simulink model "building_EXAMPLE_v1"  (R2016b)
settings: Solver=ode23tb  StartTime=-building.preruntime+8760*3600  StopTime=building.runtime+8760*3600  MaxStep=600  EnableMultiTasking=on
StartFcn:
  | tic
StopFcn:
  | toc
values from neighbouring files (symbols this model uses):
  building = create_building_automatic(building, modify, import_mode, name_XML, name_EXCEL, name_PHPP, NUMBEROFZONES)    [work_EXAMPLE_v1.m]
undefined symbols (not defined in the file or in its folder): A, B, C, cp, Dd, Dreifach, FluidMix, get_building, ID, MassFlow, p, Pressure, Qdot_C, Qdot_C_energy, Qdot_H, Qdot_H_energy, Qdot_I_electricity, Qdot_I_electricity_energy, Qdot_I_light, Qdot_I_light_energy, Qdot_I_person, Qdot_I_person_energy, Qdot_S, Qdot_S_energy, Qdot_T_ground, Qdot_T_ground_energy, Qdot_T_neighbour, Qdot_T_neighbour_energy, Qdot_T_opaque, Qdot_T_opaque_energy, Qdot_T_window, Qdot_T_window_energy, Qdot_V_infiltration, Qdot_V_infiltration_energy, Qdot_V_mech, Qdot_V_mech_energy, Qdot_V_window, Qdot_V_window_energy, rho, Tc, Temperature, Tr, Ts, Wärmeschutzglas, x_CO2, x_H2O, x_VOC
libraries: carnotUIBK x1931, carnot x83, simulink_extras x22, simulink x12
(part 34 of 35)

== system building_EXAMPLE_v1/DATALOGGER/logger_BDB/z5 ==
  BDB : Inport
  Bus Assignment : BusAssignment  AssignedSignals=Qdot_T_opaque_energy,Qdot_T_ground_energy,Qdot_T_neighbour_energy,Qdot_T_window_energy,Qdot_V_mech_energy,Qdot_V_window_energy,Qdot_V_infiltration_energy,Qdot_S_energy,Qdot_I_person_energy,Qdot_I_light_energy,Qdot_I_electricity_energy,Qdot_H_energy,Qdot_C_energy
  Bus Creator1 : BusCreator  Inputs=13
  Bus Selector1 : BusSelector  OutputSignals=z5.Qdot_T_opaque,z5.Qdot_T_ground,z5.Qdot_T_neighbour,z5.Qdot_T_window,z5.Qdot_V_mech,z5.Qdot_V_window,z5.Qdot_V_infiltration,z5.Qdot_S,z5.Qdot_I_person,z5.Qdot_I_light,z5.Qdot_I_electricity,z5.Qdot_H,z5.Qdot_C
  Constant{,1..12} (13 alike) : Constant  Value=0
  Subsystem : Subsystem
  Subsystem1 : Subsystem
  Subsystem10 : Subsystem
  Subsystem11 : Subsystem
  Subsystem12 : Subsystem
  Subsystem2 : Subsystem
  Subsystem3 : Subsystem
  Subsystem4 : Subsystem
  Subsystem5 : Subsystem
  Subsystem6 : Subsystem
  Subsystem7 : Subsystem
  Subsystem8 : Subsystem
  Subsystem9 : Subsystem
  BDBenergy : Outport
  wires:
  Constant12/1 -> Bus Creator1/13  "Qdot_C_energy"
  Constant2/1 -> Bus Creator1/3  "Qdot_T_neighbour_energy"
  Constant4/1 -> Bus Creator1/5  "Qdot_V_mech_energy"
  Constant9/1 -> Bus Creator1/10  "Qdot_I_light_energy"
  Constant1/1 -> Bus Creator1/2  "Qdot_T_ground_energy"
  Constant3/1 -> Bus Creator1/4  "Qdot_T_window_energy"
  Constant11/1 -> Bus Creator1/12  "Qdot_H_energy"
  Constant10/1 -> Bus Creator1/11  "Qdot_I_electricity_energy"
  Constant/1 -> Bus Creator1/1  "Qdot_T_opaque_energy"
  Constant8/1 -> Bus Creator1/8  "Qdot_S_energy"
  Constant7/1 -> Bus Creator1/9  "Qdot_I_person_energy"
  Constant6/1 -> Bus Creator1/7  "Qdot_V_infiltration_energy"
  BDB/1 -> Bus Selector1/1
  Constant5/1 -> Bus Creator1/6  "Qdot_V_window_energy"
  Bus Selector1/1 -> Subsystem/1(In1)  "<Qdot_T_opaque>"
  Bus Selector1/4 -> Subsystem3/1(In1)  "<Qdot_T_window>"
  Bus Selector1/3 -> Subsystem2/1(In1)  "<Qdot_T_neighbour>"
  Bus Selector1/2 -> Subsystem1/1(In1)  "<Qdot_T_ground>"
  Bus Selector1/9 -> Subsystem8/1(In1)  "<Qdot_I_person>"
  Bus Selector1/10 -> Subsystem9/1(In1)  "<Qdot_I_light>"
  Bus Selector1/11 -> Subsystem10/1(In1)  "<Qdot_I_electricity>"
  Bus Selector1/12 -> Subsystem11/1(In1)  "<Qdot_H>"
  Bus Selector1/13 -> Subsystem12/1(In1)  "<Qdot_C>"
  Bus Selector1/8 -> Subsystem7/1(In1)  "<Qdot_S>"
  Bus Selector1/7 -> Subsystem6/1(In1)  "<Qdot_V_infiltration>"
  Bus Selector1/6 -> Subsystem5/1(In1)  "<Qdot_V_window>"
  Bus Selector1/5 -> Subsystem4/1(In1)  "<Qdot_V_mech>"
  Bus Assignment/1 -> BDBenergy/1
  Bus Creator1/1 -> Bus Assignment/1
  Subsystem/1(Out1) -> Bus Assignment/2
  Subsystem12/1(Out1) -> Bus Assignment/14
  Subsystem11/1(Out1) -> Bus Assignment/13
  Subsystem10/1(Out1) -> Bus Assignment/12
  Subsystem9/1(Out1) -> Bus Assignment/11
  Subsystem8/1(Out1) -> Bus Assignment/10
  Subsystem7/1(Out1) -> Bus Assignment/9
  Subsystem6/1(Out1) -> Bus Assignment/8
  Subsystem5/1(Out1) -> Bus Assignment/7
  Subsystem4/1(Out1) -> Bus Assignment/6
  Subsystem3/1(Out1) -> Bus Assignment/5
  Subsystem2/1(Out1) -> Bus Assignment/4
  Subsystem1/1(Out1) -> Bus Assignment/3

== system building_EXAMPLE_v1/DATALOGGER/logger_BDB/z6 ==
  BDB : Inport
  Bus Assignment : BusAssignment  AssignedSignals=Qdot_T_opaque_energy,Qdot_T_ground_energy,Qdot_T_neighbour_energy,Qdot_T_window_energy,Qdot_V_mech_energy,Qdot_V_window_energy,Qdot_V_infiltration_energy,Qdot_S_energy,Qdot_I_person_energy,Qdot_I_light_energy,Qdot_I_electricity_energy,Qdot_H_energy,Qdot_C_energy
  Bus Creator1 : BusCreator  Inputs=13
  Bus Selector1 : BusSelector  OutputSignals=z6.Qdot_T_opaque,z6.Qdot_T_ground,z6.Qdot_T_neighbour,z6.Qdot_T_window,z6.Qdot_V_mech,z6.Qdot_V_window,z6.Qdot_V_infiltration,z6.Qdot_S,z6.Qdot_I_person,z6.Qdot_I_light,z6.Qdot_I_electricity,z6.Qdot_H,z6.Qdot_C
  Constant{,1..12} (13 alike) : Constant  Value=0
  Subsystem : Subsystem
  Subsystem1 : Subsystem
  Subsystem10 : Subsystem
  Subsystem11 : Subsystem
  Subsystem12 : Subsystem
  Subsystem2 : Subsystem
  Subsystem3 : Subsystem
  Subsystem4 : Subsystem
  Subsystem5 : Subsystem
  Subsystem6 : Subsystem
  Subsystem7 : Subsystem
  Subsystem8 : Subsystem
  Subsystem9 : Subsystem
  BDBenergy : Outport
  wires:
  Subsystem1/1(Out1) -> Bus Assignment/3
  Subsystem2/1(Out1) -> Bus Assignment/4
  Subsystem3/1(Out1) -> Bus Assignment/5
  Subsystem4/1(Out1) -> Bus Assignment/6
  Subsystem5/1(Out1) -> Bus Assignment/7
  Subsystem6/1(Out1) -> Bus Assignment/8
  Subsystem7/1(Out1) -> Bus Assignment/9
  Subsystem8/1(Out1) -> Bus Assignment/10
  Subsystem9/1(Out1) -> Bus Assignment/11
  Subsystem10/1(Out1) -> Bus Assignment/12
  Subsystem11/1(Out1) -> Bus Assignment/13
  Subsystem12/1(Out1) -> Bus Assignment/14
  Subsystem/1(Out1) -> Bus Assignment/2
  Bus Creator1/1 -> Bus Assignment/1
  Bus Assignment/1 -> BDBenergy/1
  Bus Selector1/5 -> Subsystem4/1(In1)  "<Qdot_V_mech>"
  Bus Selector1/6 -> Subsystem5/1(In1)  "<Qdot_V_window>"
  Bus Selector1/7 -> Subsystem6/1(In1)  "<Qdot_V_infiltration>"
  Bus Selector1/8 -> Subsystem7/1(In1)  "<Qdot_S>"
  Bus Selector1/13 -> Subsystem12/1(In1)  "<Qdot_C>"
  Bus Selector1/12 -> Subsystem11/1(In1)  "<Qdot_H>"
  Bus Selector1/11 -> Subsystem10/1(In1)  "<Qdot_I_electricity>"
  Bus Selector1/10 -> Subsystem9/1(In1)  "<Qdot_I_light>"
  Bus Selector1/9 -> Subsystem8/1(In1)  "<Qdot_I_person>"
  Bus Selector1/2 -> Subsystem1/1(In1)  "<Qdot_T_ground>"
  Bus Selector1/3 -> Subsystem2/1(In1)  "<Qdot_T_neighbour>"
  Bus Selector1/4 -> Subsystem3/1(In1)  "<Qdot_T_window>"
  Bus Selector1/1 -> Subsystem/1(In1)  "<Qdot_T_opaque>"
  Constant5/1 -> Bus Creator1/6  "Qdot_V_window_energy"
  BDB/1 -> Bus Selector1/1
  Constant6/1 -> Bus Creator1/7  "Qdot_V_infiltration_energy"
  Constant7/1 -> Bus Creator1/9  "Qdot_I_person_energy"
  Constant8/1 -> Bus Creator1/8  "Qdot_S_energy"
  Constant/1 -> Bus Creator1/1  "Qdot_T_opaque_energy"
  Constant10/1 -> Bus Creator1/11  "Qdot_I_electricity_energy"
  Constant11/1 -> Bus Creator1/12  "Qdot_H_energy"
  Constant3/1 -> Bus Creator1/4  "Qdot_T_window_energy"
  Constant1/1 -> Bus Creator1/2  "Qdot_T_ground_energy"
  Constant9/1 -> Bus Creator1/10  "Qdot_I_light_energy"
  Constant4/1 -> Bus Creator1/5  "Qdot_V_mech_energy"
  Constant2/1 -> Bus Creator1/3  "Qdot_T_neighbour_energy"
  Constant12/1 -> Bus Creator1/13  "Qdot_C_energy"

== system building_EXAMPLE_v1/DATALOGGER/logger_BDB/z7 ==
  BDB : Inport
  Bus Assignment : BusAssignment  AssignedSignals=Qdot_T_opaque_energy,Qdot_T_ground_energy,Qdot_T_neighbour_energy,Qdot_T_window_energy,Qdot_V_mech_energy,Qdot_V_window_energy,Qdot_V_infiltration_energy,Qdot_S_energy,Qdot_I_person_energy,Qdot_I_light_energy,Qdot_I_electricity_energy,Qdot_H_energy,Qdot_C_energy
  Bus Creator1 : BusCreator  Inputs=13
  Bus Selector1 : BusSelector  OutputSignals=z7.Qdot_T_opaque,z7.Qdot_T_ground,z7.Qdot_T_neighbour,z7.Qdot_T_window,z7.Qdot_V_mech,z7.Qdot_V_window,z7.Qdot_V_infiltration,z7.Qdot_S,z7.Qdot_I_person,z7.Qdot_I_light,z7.Qdot_I_electricity,z7.Qdot_H,z7.Qdot_C
  Constant{,1..12} (13 alike) : Constant  Value=0
  Subsystem : Subsystem
  Subsystem1 : Subsystem
  Subsystem10 : Subsystem
  Subsystem11 : Subsystem
  Subsystem12 : Subsystem
  Subsystem2 : Subsystem
  Subsystem3 : Subsystem
  Subsystem4 : Subsystem
  Subsystem5 : Subsystem
  Subsystem6 : Subsystem
  Subsystem7 : Subsystem
  Subsystem8 : Subsystem
  Subsystem9 : Subsystem
  BDBenergy : Outport
  wires:
  Constant12/1 -> Bus Creator1/13  "Qdot_C_energy"
  Constant2/1 -> Bus Creator1/3  "Qdot_T_neighbour_energy"
  Constant4/1 -> Bus Creator1/5  "Qdot_V_mech_energy"
  Constant9/1 -> Bus Creator1/10  "Qdot_I_light_energy"
  Constant1/1 -> Bus Creator1/2  "Qdot_T_ground_energy"
  Constant3/1 -> Bus Creator1/4  "Qdot_T_window_energy"
  Constant11/1 -> Bus Creator1/12  "Qdot_H_energy"
  Constant10/1 -> Bus Creator1/11  "Qdot_I_electricity_energy"
  Constant/1 -> Bus Creator1/1  "Qdot_T_opaque_energy"
  Constant8/1 -> Bus Creator1/8  "Qdot_S_energy"
  Constant7/1 -> Bus Creator1/9  "Qdot_I_person_energy"
  Constant6/1 -> Bus Creator1/7  "Qdot_V_infiltration_energy"
  BDB/1 -> Bus Selector1/1
  Constant5/1 -> Bus Creator1/6  "Qdot_V_window_energy"
  Bus Selector1/1 -> Subsystem/1(In1)  "<Qdot_T_opaque>"
  Bus Selector1/4 -> Subsystem3/1(In1)  "<Qdot_T_window>"
  Bus Selector1/3 -> Subsystem2/1(In1)  "<Qdot_T_neighbour>"
  Bus Selector1/2 -> Subsystem1/1(In1)  "<Qdot_T_ground>"
  Bus Selector1/9 -> Subsystem8/1(In1)  "<Qdot_I_person>"
  Bus Selector1/10 -> Subsystem9/1(In1)  "<Qdot_I_light>"
  Bus Selector1/11 -> Subsystem10/1(In1)  "<Qdot_I_electricity>"
  Bus Selector1/12 -> Subsystem11/1(In1)  "<Qdot_H>"
  Bus Selector1/13 -> Subsystem12/1(In1)  "<Qdot_C>"
  Bus Selector1/8 -> Subsystem7/1(In1)  "<Qdot_S>"
  Bus Selector1/7 -> Subsystem6/1(In1)  "<Qdot_V_infiltration>"
  Bus Selector1/6 -> Subsystem5/1(In1)  "<Qdot_V_window>"
  Bus Selector1/5 -> Subsystem4/1(In1)  "<Qdot_V_mech>"
  Bus Assignment/1 -> BDBenergy/1
  Bus Creator1/1 -> Bus Assignment/1
  Subsystem/1(Out1) -> Bus Assignment/2
  Subsystem12/1(Out1) -> Bus Assignment/14
  Subsystem11/1(Out1) -> Bus Assignment/13
  Subsystem10/1(Out1) -> Bus Assignment/12
  Subsystem9/1(Out1) -> Bus Assignment/11
  Subsystem8/1(Out1) -> Bus Assignment/10
  Subsystem7/1(Out1) -> Bus Assignment/9
  Subsystem6/1(Out1) -> Bus Assignment/8
  Subsystem5/1(Out1) -> Bus Assignment/7
  Subsystem4/1(Out1) -> Bus Assignment/6
  Subsystem3/1(Out1) -> Bus Assignment/5
  Subsystem2/1(Out1) -> Bus Assignment/4
  Subsystem1/1(Out1) -> Bus Assignment/3

== system building_EXAMPLE_v1/DATALOGGER/logger_BDB/z8 ==
  BDB : Inport
  Bus Assignment : BusAssignment  AssignedSignals=Qdot_T_opaque_energy,Qdot_T_ground_energy,Qdot_T_neighbour_energy,Qdot_T_window_energy,Qdot_V_mech_energy,Qdot_V_window_energy,Qdot_V_infiltration_energy,Qdot_S_energy,Qdot_I_person_energy,Qdot_I_light_energy,Qdot_I_electricity_energy,Qdot_H_energy,Qdot_C_energy
  Bus Creator1 : BusCreator  Inputs=13
  Bus Selector1 : BusSelector  OutputSignals=z8.Qdot_T_opaque,z8.Qdot_T_ground,z8.Qdot_T_neighbour,z8.Qdot_T_window,z8.Qdot_V_mech,z8.Qdot_V_window,z8.Qdot_V_infiltration,z8.Qdot_S,z8.Qdot_I_person,z8.Qdot_I_light,z8.Qdot_I_electricity,z8.Qdot_H,z8.Qdot_C
  Constant{,1..12} (13 alike) : Constant  Value=0
  Subsystem : Subsystem
  Subsystem1 : Subsystem
  Subsystem10 : Subsystem
  Subsystem11 : Subsystem
  Subsystem12 : Subsystem
  Subsystem2 : Subsystem
  Subsystem3 : Subsystem
  Subsystem4 : Subsystem
  Subsystem5 : Subsystem
  Subsystem6 : Subsystem
  Subsystem7 : Subsystem
  Subsystem8 : Subsystem
  Subsystem9 : Subsystem
  BDBenergy : Outport
  wires:
  Subsystem1/1(Out1) -> Bus Assignment/3
  Subsystem2/1(Out1) -> Bus Assignment/4
  Subsystem3/1(Out1) -> Bus Assignment/5
  Subsystem4/1(Out1) -> Bus Assignment/6
  Subsystem5/1(Out1) -> Bus Assignment/7
  Subsystem6/1(Out1) -> Bus Assignment/8
  Subsystem7/1(Out1) -> Bus Assignment/9
  Subsystem8/1(Out1) -> Bus Assignment/10
  Subsystem9/1(Out1) -> Bus Assignment/11
  Subsystem10/1(Out1) -> Bus Assignment/12
  Subsystem11/1(Out1) -> Bus Assignment/13
  Subsystem12/1(Out1) -> Bus Assignment/14
  Subsystem/1(Out1) -> Bus Assignment/2
  Bus Creator1/1 -> Bus Assignment/1
  Bus Assignment/1 -> BDBenergy/1
  Bus Selector1/5 -> Subsystem4/1(In1)  "<Qdot_V_mech>"
  Bus Selector1/6 -> Subsystem5/1(In1)  "<Qdot_V_window>"
  Bus Selector1/7 -> Subsystem6/1(In1)  "<Qdot_V_infiltration>"
  Bus Selector1/8 -> Subsystem7/1(In1)  "<Qdot_S>"
  Bus Selector1/13 -> Subsystem12/1(In1)  "<Qdot_C>"
  Bus Selector1/12 -> Subsystem11/1(In1)  "<Qdot_H>"
  Bus Selector1/11 -> Subsystem10/1(In1)  "<Qdot_I_electricity>"
  Bus Selector1/10 -> Subsystem9/1(In1)  "<Qdot_I_light>"
  Bus Selector1/9 -> Subsystem8/1(In1)  "<Qdot_I_person>"
  Bus Selector1/2 -> Subsystem1/1(In1)  "<Qdot_T_ground>"
  Bus Selector1/3 -> Subsystem2/1(In1)  "<Qdot_T_neighbour>"
  Bus Selector1/4 -> Subsystem3/1(In1)  "<Qdot_T_window>"
  Bus Selector1/1 -> Subsystem/1(In1)  "<Qdot_T_opaque>"
  Constant5/1 -> Bus Creator1/6  "Qdot_V_window_energy"
  BDB/1 -> Bus Selector1/1
  Constant6/1 -> Bus Creator1/7  "Qdot_V_infiltration_energy"
  Constant7/1 -> Bus Creator1/9  "Qdot_I_person_energy"
  Constant8/1 -> Bus Creator1/8  "Qdot_S_energy"
  Constant/1 -> Bus Creator1/1  "Qdot_T_opaque_energy"
  Constant10/1 -> Bus Creator1/11  "Qdot_I_electricity_energy"
  Constant11/1 -> Bus Creator1/12  "Qdot_H_energy"
  Constant3/1 -> Bus Creator1/4  "Qdot_T_window_energy"
  Constant1/1 -> Bus Creator1/2  "Qdot_T_ground_energy"
  Constant9/1 -> Bus Creator1/10  "Qdot_I_light_energy"
  Constant4/1 -> Bus Creator1/5  "Qdot_V_mech_energy"
  Constant2/1 -> Bus Creator1/3  "Qdot_T_neighbour_energy"
  Constant12/1 -> Bus Creator1/13  "Qdot_C_energy"

== system building_EXAMPLE_v1/DATALOGGER/logger_BDB/z9 ==
  BDB : Inport
  Bus Assignment : BusAssignment  AssignedSignals=Qdot_T_opaque_energy,Qdot_T_ground_energy,Qdot_T_neighbour_energy,Qdot_T_window_energy,Qdot_V_mech_energy,Qdot_V_window_energy,Qdot_V_infiltration_energy,Qdot_S_energy,Qdot_I_person_energy,Qdot_I_light_energy,Qdot_I_electricity_energy,Qdot_H_energy,Qdot_C_energy
  Bus Creator1 : BusCreator  Inputs=13
  Bus Selector1 : BusSelector  OutputSignals=z9.Qdot_T_opaque,z9.Qdot_T_ground,z9.Qdot_T_neighbour,z9.Qdot_T_window,z9.Qdot_V_mech,z9.Qdot_V_window,z9.Qdot_V_infiltration,z9.Qdot_S,z9.Qdot_I_person,z9.Qdot_I_light,z9.Qdot_I_electricity,z9.Qdot_H,z9.Qdot_C
  Constant{,1..12} (13 alike) : Constant  Value=0
  Subsystem : Subsystem
  Subsystem1 : Subsystem
  Subsystem10 : Subsystem
  Subsystem11 : Subsystem
  Subsystem12 : Subsystem
  Subsystem2 : Subsystem
  Subsystem3 : Subsystem
  Subsystem4 : Subsystem
  Subsystem5 : Subsystem
  Subsystem6 : Subsystem
  Subsystem7 : Subsystem
  Subsystem8 : Subsystem
  Subsystem9 : Subsystem
  BDBenergy : Outport
  wires:
  Constant12/1 -> Bus Creator1/13  "Qdot_C_energy"
  Constant2/1 -> Bus Creator1/3  "Qdot_T_neighbour_energy"
  Constant4/1 -> Bus Creator1/5  "Qdot_V_mech_energy"
  Constant9/1 -> Bus Creator1/10  "Qdot_I_light_energy"
  Constant1/1 -> Bus Creator1/2  "Qdot_T_ground_energy"
  Constant3/1 -> Bus Creator1/4  "Qdot_T_window_energy"
  Constant11/1 -> Bus Creator1/12  "Qdot_H_energy"
  Constant10/1 -> Bus Creator1/11  "Qdot_I_electricity_energy"
  Constant/1 -> Bus Creator1/1  "Qdot_T_opaque_energy"
  Constant8/1 -> Bus Creator1/8  "Qdot_S_energy"
  Constant7/1 -> Bus Creator1/9  "Qdot_I_person_energy"
  Constant6/1 -> Bus Creator1/7  "Qdot_V_infiltration_energy"
  BDB/1 -> Bus Selector1/1
  Constant5/1 -> Bus Creator1/6  "Qdot_V_window_energy"
  Bus Selector1/1 -> Subsystem/1(In1)  "<Qdot_T_opaque>"
  Bus Selector1/4 -> Subsystem3/1(In1)  "<Qdot_T_window>"
  Bus Selector1/3 -> Subsystem2/1(In1)  "<Qdot_T_neighbour>"
  Bus Selector1/2 -> Subsystem1/1(In1)  "<Qdot_T_ground>"
  Bus Selector1/9 -> Subsystem8/1(In1)  "<Qdot_I_person>"
  Bus Selector1/10 -> Subsystem9/1(In1)  "<Qdot_I_light>"
  Bus Selector1/11 -> Subsystem10/1(In1)  "<Qdot_I_electricity>"
  Bus Selector1/12 -> Subsystem11/1(In1)  "<Qdot_H>"
  Bus Selector1/13 -> Subsystem12/1(In1)  "<Qdot_C>"
  Bus Selector1/8 -> Subsystem7/1(In1)  "<Qdot_S>"
  Bus Selector1/7 -> Subsystem6/1(In1)  "<Qdot_V_infiltration>"
  Bus Selector1/6 -> Subsystem5/1(In1)  "<Qdot_V_window>"
  Bus Selector1/5 -> Subsystem4/1(In1)  "<Qdot_V_mech>"
  Bus Assignment/1 -> BDBenergy/1
  Bus Creator1/1 -> Bus Assignment/1
  Subsystem/1(Out1) -> Bus Assignment/2
  Subsystem12/1(Out1) -> Bus Assignment/14
  Subsystem11/1(Out1) -> Bus Assignment/13
  Subsystem10/1(Out1) -> Bus Assignment/12
  Subsystem9/1(Out1) -> Bus Assignment/11
  Subsystem8/1(Out1) -> Bus Assignment/10
  Subsystem7/1(Out1) -> Bus Assignment/9
  Subsystem6/1(Out1) -> Bus Assignment/8
  Subsystem5/1(Out1) -> Bus Assignment/7
  Subsystem4/1(Out1) -> Bus Assignment/6
  Subsystem3/1(Out1) -> Bus Assignment/5
  Subsystem2/1(Out1) -> Bus Assignment/4
  Subsystem1/1(Out1) -> Bus Assignment/3

== system building_EXAMPLE_v1/HVAC PKOM4/HR/calc_h ==
  theta : Inport
  x : Inport  Port=2
  1.006 : Gain  Gain=1.006
  1.86 : Gain  Gain=1.86
  2500 : Bias  Bias=2500
  Add3 : Sum
  Product : Product
  "kJ -> J" : Gain  Gain=1000
  h : Outport
  wires:
  2500/1 -> Product/1
  1.006/1 -> Add3/1
  Add3/1 -> "kJ -> J"/1
  Product/1 -> Add3/2
  1.86/1 -> 2500/1
  x/1 -> Product/2
  theta/1 -> 1.86/1, 1.006/1
  "kJ -> J"/1 -> h/1

== system building_EXAMPLE_v1/HVAC PKOM4/HR unit/calc_h ==
  theta : Inport
  x : Inport  Port=2
  1.006 : Gain  Gain=1.006
  1.86 : Gain  Gain=1.86
  2500 : Bias  Bias=2500
  Add3 : Sum
  Product : Product
  "kJ -> J" : Gain  Gain=1000
  h : Outport
  wires:
  2500/1 -> Product/1
  1.006/1 -> Add3/1
  Add3/1 -> "kJ -> J"/1
  Product/1 -> Add3/2
  1.86/1 -> 2500/1
  x/1 -> Product/2
  theta/1 -> 1.86/1, 1.006/1
  "kJ -> J"/1 -> h/1

== system building_EXAMPLE_v1/HVAC PKOM4/HR+MR/calc_h ==
  theta : Inport
  x : Inport  Port=2
  1.006 : Gain  Gain=1.006
  1.86 : Gain  Gain=1.86
  2500 : Bias  Bias=2500
  Add3 : Sum
  Product : Product
  "kJ -> J" : Gain  Gain=1000
  h : Outport
  wires:
  "kJ -> J"/1 -> h/1
  theta/1 -> 1.006/1, 1.86/1
  x/1 -> Product/2
  1.86/1 -> 2500/1
  Product/1 -> Add3/2
  Add3/1 -> "kJ -> J"/1
  1.006/1 -> Add3/1
  2500/1 -> Product/1

== system building_EXAMPLE_v1/HVAC PKOM4/HR+MR unit/calc_h ==
  theta : Inport
  x : Inport  Port=2
  1.006 : Gain  Gain=1.006
  1.86 : Gain  Gain=1.86
  2500 : Bias  Bias=2500
  Add3 : Sum
  Product : Product
  "kJ -> J" : Gain  Gain=1000
  h : Outport
  wires:
  "kJ -> J"/1 -> h/1
  theta/1 -> 1.006/1, 1.86/1
  x/1 -> Product/2
  1.86/1 -> 2500/1
  Product/1 -> Add3/2
  Add3/1 -> "kJ -> J"/1
  1.006/1 -> Add3/1
  2500/1 -> Product/1

== system building_EXAMPLE_v1/HVAC PKOM4/electrical heater 1/Transfer Fcn (with initial states) ==
  In1 : Inport
  State Space : StateSpace  A=A  B=B  C=C  D=Dd  X0=X0
  Out1 : Outport  InitialOutput=0
  wires:
  State Space/1 -> Out1/1
  In1/1 -> State Space/1

== system building_EXAMPLE_v1/HVAC PKOM4/electrical heater 1/Transfer Fcn (with initial states)6 ==
  In1 : Inport
  State Space : StateSpace  A=A  B=B  C=C  D=Dd  X0=X0
  Out1 : Outport  InitialOutput=0
  wires:
  In1/1 -> State Space/1
  State Space/1 -> Out1/1

== system building_EXAMPLE_v1/HVAC PKOM4/electrical heater 2/Transfer Fcn (with initial states) ==
  In1 : Inport
  State Space : StateSpace  A=A  B=B  C=C  D=Dd  X0=X0
  Out1 : Outport  InitialOutput=0
  wires:
  In1/1 -> State Space/1
  State Space/1 -> Out1/1

== system building_EXAMPLE_v1/HVAC PKOM4/electrical heater 2/Transfer Fcn (with initial states)6 ==
  In1 : Inport
  State Space : StateSpace  A=A  B=B  C=C  D=Dd  X0=X0
  Out1 : Outport  InitialOutput=0
  wires:
  State Space/1 -> Out1/1
  In1/1 -> State Space/1

== system building_EXAMPLE_v1/HVAC PKOM4/electrical heater 3/Transfer Fcn (with initial states) ==
  In1 : Inport
  State Space : StateSpace  A=A  B=B  C=C  D=Dd  X0=X0
  Out1 : Outport  InitialOutput=0
  wires:
  State Space/1 -> Out1/1
  In1/1 -> State Space/1

== system building_EXAMPLE_v1/HVAC PKOM4/electrical heater 3/Transfer Fcn (with initial states)6 ==
  In1 : Inport
  State Space : StateSpace  A=A  B=B  C=C  D=Dd  X0=X0
  Out1 : Outport  InitialOutput=0
  wires:
  In1/1 -> State Space/1
  State Space/1 -> Out1/1

== system building_EXAMPLE_v1/HVAC PKOM4/electrical heater 4 CONVECTOR/Transfer Fcn (with initial states) ==
  In1 : Inport
  State Space : StateSpace  A=A  B=B  C=C  D=Dd  X0=X0
  Out1 : Outport  InitialOutput=0
  wires:
  In1/1 -> State Space/1
  State Space/1 -> Out1/1

== system building_EXAMPLE_v1/HVAC PKOM4/electrical heater 4 CONVECTOR/Transfer Fcn (with initial states)6 ==
  In1 : Inport
  State Space : StateSpace  A=A  B=B  C=C  D=Dd  X0=X0
  Out1 : Outport  InitialOutput=0
  wires:
  State Space/1 -> Out1/1
  In1/1 -> State Space/1

== system building_EXAMPLE_v1/HVAC PKOM4/electrical heater 5/Transfer Fcn (with initial states) ==
  In1 : Inport
  State Space : StateSpace  A=A  B=B  C=C  D=Dd  X0=X0
  Out1 : Outport  InitialOutput=0
  wires:
  State Space/1 -> Out1/1
  In1/1 -> State Space/1

== system building_EXAMPLE_v1/HVAC PKOM4/electrical heater 5/Transfer Fcn (with initial states)6 ==
  In1 : Inport
  State Space : StateSpace  A=A  B=B  C=C  D=Dd  X0=X0
  Out1 : Outport  InitialOutput=0
  wires:
  In1/1 -> State Space/1
  State Space/1 -> Out1/1

== system building_EXAMPLE_v1/HVAC PKOM4/electrical heater 6/Transfer Fcn (with initial states) ==
  In1 : Inport
  State Space : StateSpace  A=A  B=B  C=C  D=Dd  X0=X0
  Out1 : Outport  InitialOutput=0
  wires:
  In1/1 -> State Space/1
  State Space/1 -> Out1/1

== system building_EXAMPLE_v1/HVAC PKOM4/electrical heater 6/Transfer Fcn (with initial states)6 ==
  In1 : Inport
  State Space : StateSpace  A=A  B=B  C=C  D=Dd  X0=X0
  Out1 : Outport  InitialOutput=0
  wires:
  State Space/1 -> Out1/1
  In1/1 -> State Space/1

== system building_EXAMPLE_v1/HVAC PKOM4/electrical heater 7/Transfer Fcn (with initial states) ==
  In1 : Inport
  State Space : StateSpace  A=A  B=B  C=C  D=Dd  X0=X0
  Out1 : Outport  InitialOutput=0
  wires:
  State Space/1 -> Out1/1
  In1/1 -> State Space/1

== system building_EXAMPLE_v1/HVAC PKOM4/electrical heater 7/Transfer Fcn (with initial states)6 ==
  In1 : Inport
  State Space : StateSpace  A=A  B=B  C=C  D=Dd  X0=X0
  Out1 : Outport  InitialOutput=0
  wires:
  In1/1 -> State Space/1
  State Space/1 -> Out1/1

== system building_EXAMPLE_v1/HVAC PKOM4/heatpump heating/calc_Pel_compressor ==
  u : Inport
  Selector : Selector  InputPortWidth=2  IndexOptions=Index vector (dialog)  Indices=[2]  OutputSizes=1
  lu : Fcn  Expr=pol.p00 + pol.p10*u(1) + pol.p01*u(2) + pol.p20*u(1)^2 + pol.p11*u(1)*u(2) + pol.p02*u(2)^2 + pol.p30*u(1)^3 + pol.p21*u(1)^2*u(2) + pol.p12*u(1)*u(2)^2 + pol.p03*u(2)^3 + pol.p31*u(1)^3*u(2) + pol.p22*u(1)^2*u(2)^2 + pol.p13*u(1)*u(2)^3 + pol.p04*u(2)^4
  no power : Constant  Value=0
  on/off HP : Switch  Threshold=1
  y : Outport
  wires:
  u/1 -> Selector/1, lu/1
  Selector/1 -> on/off HP/2
  lu/1 -> on/off HP/1
  on/off HP/1 -> y/1
  no power/1 -> on/off HP/3

== system building_EXAMPLE_v1/HVAC PKOM4/heatpump heating/calc_Pel_compressor_useable ==
  u : Inport
  Selector : Selector  InputPortWidth=2  IndexOptions=Index vector (dialog)  Indices=[2]  OutputSizes=1
  lu : Fcn  Expr=pol.p00 + pol.p10*u(1) + pol.p01*u(2) + pol.p20*u(1)^2 + pol.p11*u(1)*u(2) + pol.p02*u(2)^2 + pol.p30*u(1)^3 + pol.p21*u(1)^2*u(2) + pol.p12*u(1)*u(2)^2 + pol.p03*u(2)^3 + pol.p31*u(1)^3*u(2) + pol.p22*u(1)^2*u(2)^2 + pol.p13*u(1)*u(2)^3 + pol.p04*u(2)^4
  no power : Constant  Value=0
  on/off HP : Switch  Threshold=1
  y : Outport
  wires:
  no power/1 -> on/off HP/3
  on/off HP/1 -> y/1
  lu/1 -> on/off HP/1
  Selector/1 -> on/off HP/2
  u/1 -> lu/1, Selector/1

== system building_EXAMPLE_v1/HVAC PKOM4/heatpump heating/calc_Qdot_sup ==
  u : Inport
  Selector : Selector  InputPortWidth=2  IndexOptions=Index vector (dialog)  Indices=[2]  OutputSizes=1
  lu : Fcn  Expr=pol.p00 + pol.p10*u(1) + pol.p01*u(2) + pol.p20*u(1)^2 + pol.p11*u(1)*u(2) + pol.p02*u(2)^2 + pol.p30*u(1)^3 + pol.p21*u(1)^2*u(2) + pol.p12*u(1)*u(2)^2 + pol.p03*u(2)^3 + pol.p31*u(1)^3*u(2) + pol.p22*u(1)^2*u(2)^2 + pol.p13*u(1)*u(2)^3 + pol.p04*u(2)^4
  no power : Constant  Value=0
  on/off HP : Switch  Threshold=1
  y : Outport
  wires:
  u/1 -> Selector/1, lu/1
  Selector/1 -> on/off HP/2
  lu/1 -> on/off HP/1
  on/off HP/1 -> y/1
  no power/1 -> on/off HP/3

== system building_EXAMPLE_v1/HVAC PKOM4/heatpump heating/calc_deicing ==
  u : Inport
  Demux : Demux  Outputs=2
  Gain3 : Gain  Gain=60
  Mux2 : Mux  Inputs=2
  limit deicing time : Saturate  UpperLimit=5*60*60  LowerLimit=60*60
  limit h : Saturate  UpperLimit=inf  LowerLimit=15000
  lu : Fcn  Expr=pol.p00 + pol.p10*u(1) + pol.p01*u(2) + pol.p20*u(1)^2 + pol.p11*u(1)*u(2) + pol.p02*u(2)^2 + pol.p30*u(1)^3 + pol.p21*u(1)^2*u(2) + pol.p12*u(1)*u(2)^2 + pol.p03*u(2)^3 + pol.p31*u(1)^3*u(2) + pol.p22*u(1)^2*u(2)^2 + pol.p13*u(1)*u(2)^3 + pol.p04*u(2)^4
  deicing time : Outport
  wires:
  Mux2/1 -> lu/1
  Demux/1 -> limit h/1
  Demux/2 -> Mux2/2
  u/1 -> Demux/1
  limit h/1 -> Mux2/1
  Gain3/1 -> limit deicing time/1
  lu/1 -> Gain3/1
  limit deicing time/1 -> deicing time/1

== system building_EXAMPLE_v1/HVAC pipes/Pipes_inlet/THB_split3 ==
  THBin : Inport
  Add1 : Sum
  Bus Assignment : BusAssignment  AssignedSignals=MassFlow
  Bus Assignment1 : BusAssignment  AssignedSignals=ID,MassFlow
  Bus Selector : BusSelector  OutputSignals=ID,MassFlow
  Constant : Constant
  Gain1 : Gain  Gain=(hvac.zone_5.perc_Vdot_tot + hvac.zone_6.perc_Vdot_tot)
  Gain2 : Gain  Gain=hvac.zone_2.perc_Vdot_tot
  THB1out : Outport  InitialOutput=0
  THB2out : Outport  Port=2  InitialOutput=0
  wires:
  THBin/1 -> Bus Selector/1, Bus Assignment1/1, Bus Assignment/1
  Bus Assignment/1 -> THB1out/1
  Bus Assignment1/1 -> THB2out/1
  Constant/1 -> Add1/1
  Bus Selector/2 -> Gain2/1, Gain1/1  "<MassFlow>"
  Gain2/1 -> Bus Assignment1/3
  Gain1/1 -> Bus Assignment/2
  Bus Selector/1 -> Add1/2  "<ID>"
  Add1/1 -> Bus Assignment1/2

== system building_EXAMPLE_v1/HVAC pipes/Pipes_inlet/THB_split4 ==
  THBin : Inport
  Add1 : Sum
  Bus Assignment2 : BusAssignment  AssignedSignals=MassFlow
  Bus Assignment3 : BusAssignment  AssignedSignals=ID,MassFlow
  Bus Selector : BusSelector  OutputSignals=ID,MassFlow
  Constant1 : Constant
  Gain2 : Gain  Gain=(hvac.zone_5.perc_Vdot_tot)/(1-hvac.zone_2.perc_Vdot_tot)
  Gain3 : Gain  Gain=(hvac.zone_6.perc_Vdot_tot)/(1-hvac.zone_2.perc_Vdot_tot)
  THB1out : Outport  InitialOutput=0
  THB2out : Outport  Port=2  InitialOutput=0
  wires:
  THBin/1 -> Bus Selector/1, Bus Assignment3/1, Bus Assignment2/1
  Bus Assignment2/1 -> THB1out/1
  Bus Assignment3/1 -> THB2out/1
  Constant1/1 -> Add1/1
  Bus Selector/2 -> Gain3/1, Gain2/1  "<MassFlow>"
  Gain3/1 -> Bus Assignment3/3
  Gain2/1 -> Bus Assignment2/2
  Bus Selector/1 -> Add1/2  "<ID>"
  Add1/1 -> Bus Assignment3/2

== system building_EXAMPLE_v1/HVAC pipes/Pipes_outlet/Subsystem ==
  T_bad : Inport
  rho_bad : Inport  Port=2
  P_bad : Inport  Port=3
  x_H2O_bad : Inport  Port=4
  T_kueche : Inport  Port=5
  rho_kueche : Inport  Port=6
  P_kueche : Inport  Port=7
  x_H2O_kueche : Inport  Port=8
  Gain1 : Gain  Gain=hvac.zone_4.perc_Vdot_tot
  Gain10 : Gain  Gain=hvac.zone_1.perc_Vdot_tot
  THV2THB : carnot/Toolbox/THV2THB
  THV2THB1 : carnot/Toolbox/THV2THB
  Vdot_Total : Constant  Value=hvac.Vdot_tot
  kg/s : Gain  Gain=1/3600
  kg/s1 : Gain  Gain=1/3600
  mdot : Product  RndMeth=Zero
  mdot1 : Product  RndMeth=Zero
  supply : Subsystem  AncestorBlock=carnot/misc/create_THV  mask(create THV){p=1e5, fluid=air, mix=0, dia=0.125}
      mask prompts: p "pressure [Pa]"; mix "fluid mixture [0..1]"; dia "diameter [m]"
      mask help: Block to create a THV vector with the variable input T and mdot. The other value can be set as constants in the mask.
      mask init:
      | mix = min(1, max(0, mix));
      | dia = max(dia, 0.001);
      mask Help: eval('man (''create_THV'')')
      mask TypeOptions fluid: water | air | cotton_oil | silicone_oil | water_glycol_mix | tyfocor_LS
  supply1 : Subsystem  AncestorBlock=carnot/misc/create_THV  mask(create THV){p=1e5, fluid=air, mix=0, dia=0.125}
      mask prompts: p "pressure [Pa]"; mix "fluid mixture [0..1]"; dia "diameter [m]"
      mask help: Block to create a THV vector with the variable input T and mdot. The other value can be set as constants in the mask.
      mask init:
      | mix = min(1, max(0, mix));
      | dia = max(dia, 0.001);
      mask Help: eval('man (''create_THV'')')
      mask TypeOptions fluid: water | air | cotton_oil | silicone_oil | water_glycol_mix | tyfocor_LS
  THB_bad : Outport  InitialOutput=0
  THB_kuche : Outport  Port=2  InitialOutput=0
  wires:
  x_H2O_bad/1 -> supply/4(mix)
  T_bad/1 -> supply/1(T)
  kg/s1/1 -> supply/2(mdot)
  Gain1/1 -> mdot1/1
  rho_bad/1 -> mdot1/2
  P_bad/1 -> supply/3(p)
  mdot1/1 -> kg/s1/1
  Gain10/1 -> mdot/1
  rho_kueche/1 -> mdot/2
  mdot/1 -> kg/s/1
  x_H2O_kueche/1 -> supply1/4(mix)
  T_kueche/1 -> supply1/1(T)
  kg/s/1 -> supply1/2(mdot)
  P_kueche/1 -> supply1/3(p)
  supply/1(THV) -> THV2THB/1
  THV2THB/1 -> THB_bad/1
  supply1/1(THV) -> THV2THB1/1
  THV2THB1/1 -> THB_kuche/1
  Vdot_Total/1 -> Gain10/1, Gain1/1

== system building_EXAMPLE_v1/HVAC pipes/Pipes_outlet/mix ==
  THB_1 : Inport
  THB_2 : Inport  Port=2
  Add{,1..3} (4 alike) : Sum
  Bus Assignment : BusAssignment  AssignedSignals=Temperature,MassFlow,Pressure,FluidMix
  Bus Selector : BusSelector  OutputSignals=Temperature,MassFlow,Pressure,FluidMix
  Bus Selector2 : BusSelector  OutputSignals=Temperature,MassFlow,Pressure,FluidMix
  Divide : Product  Inputs=*/
  Divide1 : Product  Inputs=*/
  Divide2 : Product  Inputs=*/
  Product{,1..5} (6 alike) : Product
  THB_common : Outport
  wires:
  Add/1 -> Divide/1
  Product1/1 -> Add/2
  Product/1 -> Add/1
  THB_1/1 -> Bus Selector/1
  Add2/1 -> Divide1/1
  Product2/1 -> Add2/1
  Product3/1 -> Add2/2
  THB_2/1 -> Bus Selector2/1, Bus Assignment/1
  Product4/1 -> Add3/1
  Product5/1 -> Add3/2
  Add3/1 -> Divide2/1
  Add1/1 -> Divide/2, Divide2/2, Divide1/2, Bus Assignment/3
  Bus Assignment/1 -> THB_common/1
  Divide2/1 -> Bus Assignment/5
  Divide1/1 -> Bus Assignment/4
  Divide/1 -> Bus Assignment/2
  Bus Selector/1 -> Product/1  "<Temperature>"
  Bus Selector2/1 -> Product1/1  "<Temperature>"
  Bus Selector/3 -> Product2/2  "<Pressure>"
  Bus Selector2/3 -> Product3/2  "<Pressure>"
  Bus Selector/4 -> Product4/2  "<FluidMix>"
  Bus Selector2/4 -> Product5/2  "<FluidMix>"
  Bus Selector/2 -> Product4/1, Product2/1, Add1/1, Product/2  "<MassFlow>"
  Bus Selector2/2 -> Product3/1, Product5/1, Add1/2, Product1/2  "<MassFlow>"

== system building_EXAMPLE_v1/HVAC pipes/ventilation_outlet1_z1/create_THB ==
  mdot : Inport
  T : Inport  Port=2
  p : Inport  Port=3
  mix : Inport  Port=4
  THB_set_T : carnot/Source/Simple/THB_set_T
  THB_set_mdot : carnot/Source/Simple/THB_set_mdot
  THB_set_mix : Subsystem  InitFcn=load('THB.mat');  mask(set temperature in THB){}
      mask help: Set a variable temperature in the thermo-hydraulic bus.
      mask Help: web(['file:///' fullfile(path_carnot('help'),'THB_set_T.html')],'-helpbrowser')
  THB_set_p : Subsystem  InitFcn=load('THB.mat');  mask(set temperature in THB){}
      mask help: Set a variable temperature in the thermo-hydraulic bus.
      mask Help: web(['file:///' fullfile(path_carnot('help'),'THB_set_T.html')],'-helpbrowser')
  basic_THB : carnot/Basic/Hydraulics/basic_THB  t=20  mdot=0  p=1e5  ID=1  fluid=2  mix=0  dia=0.125  hgt=0
  THB : Outport
  wires:
  T/1 -> THB_set_T/2
  THB_set_mdot/1 -> THB_set_T/1
  mdot/1 -> THB_set_mdot/2
  basic_THB/1 -> THB_set_mdot/1
  THB_set_T/1 -> THB_set_p/1(THB_in)
  THB_set_p/1(THB) -> THB_set_mix/1(THB_in)
  THB_set_mix/1(THB) -> THB/1
  p/1 -> THB_set_p/2(p)
  mix/1 -> THB_set_mix/2(mix)

== system building_EXAMPLE_v1/HVAC pipes/ventilation_outlet1_z10/create_THB ==
  mdot : Inport
  T : Inport  Port=2
  p : Inport  Port=3
  mix : Inport  Port=4
  THB_set_T : carnot/Source/Simple/THB_set_T
  THB_set_mdot : carnot/Source/Simple/THB_set_mdot
  THB_set_mix : Subsystem  InitFcn=load('THB.mat');  mask(set temperature in THB){}
      mask help: Set a variable temperature in the thermo-hydraulic bus.
      mask Help: web(['file:///' fullfile(path_carnot('help'),'THB_set_T.html')],'-helpbrowser')
  THB_set_p : Subsystem  InitFcn=load('THB.mat');  mask(set temperature in THB){}
      mask help: Set a variable temperature in the thermo-hydraulic bus.
      mask Help: web(['file:///' fullfile(path_carnot('help'),'THB_set_T.html')],'-helpbrowser')
  basic_THB : carnot/Basic/Hydraulics/basic_THB  t=20  mdot=0  p=1e5  ID=1  fluid=2  mix=0  dia=0.125  hgt=0
  THB : Outport
  wires:
  T/1 -> THB_set_T/2
  THB_set_mdot/1 -> THB_set_T/1
  mdot/1 -> THB_set_mdot/2
  basic_THB/1 -> THB_set_mdot/1
  THB_set_T/1 -> THB_set_p/1(THB_in)
  THB_set_p/1(THB) -> THB_set_mix/1(THB_in)
  THB_set_mix/1(THB) -> THB/1
  p/1 -> THB_set_p/2(p)
  mix/1 -> THB_set_mix/2(mix)

== system building_EXAMPLE_v1/HVAC pipes/ventilation_outlet1_z2/create_THB ==
  mdot : Inport
  T : Inport  Port=2
  p : Inport  Port=3
  mix : Inport  Port=4
  THB_set_T : carnot/Source/Simple/THB_set_T
  THB_set_mdot : carnot/Source/Simple/THB_set_mdot
  THB_set_mix : Subsystem  InitFcn=load('THB.mat');  mask(set temperature in THB){}
      mask help: Set a variable temperature in the thermo-hydraulic bus.
      mask Help: web(['file:///' fullfile(path_carnot('help'),'THB_set_T.html')],'-helpbrowser')
  THB_set_p : Subsystem  InitFcn=load('THB.mat');  mask(set temperature in THB){}
      mask help: Set a variable temperature in the thermo-hydraulic bus.
      mask Help: web(['file:///' fullfile(path_carnot('help'),'THB_set_T.html')],'-helpbrowser')
  basic_THB : carnot/Basic/Hydraulics/basic_THB  t=20  mdot=0  p=1e5  ID=1  fluid=2  mix=0  dia=0.125  hgt=0
  THB : Outport
  wires:
  T/1 -> THB_set_T/2
  THB_set_mdot/1 -> THB_set_T/1
  mdot/1 -> THB_set_mdot/2
  basic_THB/1 -> THB_set_mdot/1
  THB_set_T/1 -> THB_set_p/1(THB_in)
  THB_set_p/1(THB) -> THB_set_mix/1(THB_in)
  THB_set_mix/1(THB) -> THB/1
  p/1 -> THB_set_p/2(p)
  mix/1 -> THB_set_mix/2(mix)

== system building_EXAMPLE_v1/HVAC pipes/ventilation_outlet1_z3/create_THB ==
  mdot : Inport
  T : Inport  Port=2
  p : Inport  Port=3
  mix : Inport  Port=4
  THB_set_T : carnot/Source/Simple/THB_set_T
  THB_set_mdot : carnot/Source/Simple/THB_set_mdot
  THB_set_mix : Subsystem  InitFcn=load('THB.mat');  mask(set temperature in THB){}
      mask help: Set a variable temperature in the thermo-hydraulic bus.
      mask Help: web(['file:///' fullfile(path_carnot('help'),'THB_set_T.html')],'-helpbrowser')
  THB_set_p : Subsystem  InitFcn=load('THB.mat');  mask(set temperature in THB){}
      mask help: Set a variable temperature in the thermo-hydraulic bus.
      mask Help: web(['file:///' fullfile(path_carnot('help'),'THB_set_T.html')],'-helpbrowser')
  basic_THB : carnot/Basic/Hydraulics/basic_THB  t=20  mdot=0  p=1e5  ID=1  fluid=2  mix=0  dia=0.125  hgt=0
  THB : Outport
  wires:
  T/1 -> THB_set_T/2
  THB_set_mdot/1 -> THB_set_T/1
  mdot/1 -> THB_set_mdot/2
  basic_THB/1 -> THB_set_mdot/1
  THB_set_T/1 -> THB_set_p/1(THB_in)
  THB_set_p/1(THB) -> THB_set_mix/1(THB_in)
  THB_set_mix/1(THB) -> THB/1
  p/1 -> THB_set_p/2(p)
  mix/1 -> THB_set_mix/2(mix)

== system building_EXAMPLE_v1/HVAC pipes/ventilation_outlet1_z4/create_THB ==
  mdot : Inport
  T : Inport  Port=2
  p : Inport  Port=3
  mix : Inport  Port=4
  THB_set_T : carnot/Source/Simple/THB_set_T
  THB_set_mdot : carnot/Source/Simple/THB_set_mdot
  THB_set_mix : Subsystem  InitFcn=load('THB.mat');  mask(set temperature in THB){}
      mask help: Set a variable temperature in the thermo-hydraulic bus.
      mask Help: web(['file:///' fullfile(path_carnot('help'),'THB_set_T.html')],'-helpbrowser')
  THB_set_p : Subsystem  InitFcn=load('THB.mat');  mask(set temperature in THB){}
      mask help: Set a variable temperature in the thermo-hydraulic bus.
      mask Help: web(['file:///' fullfile(path_carnot('help'),'THB_set_T.html')],'-helpbrowser')
  basic_THB : carnot/Basic/Hydraulics/basic_THB  t=20  mdot=0  p=1e5  ID=1  fluid=2  mix=0  dia=0.125  hgt=0
  THB : Outport
  wires:
  T/1 -> THB_set_T/2
  THB_set_mdot/1 -> THB_set_T/1
  mdot/1 -> THB_set_mdot/2
  basic_THB/1 -> THB_set_mdot/1
  THB_set_T/1 -> THB_set_p/1(THB_in)
  THB_set_p/1(THB) -> THB_set_mix/1(THB_in)
  THB_set_mix/1(THB) -> THB/1
  p/1 -> THB_set_p/2(p)
  mix/1 -> THB_set_mix/2(mix)

== system building_EXAMPLE_v1/HVAC pipes/ventilation_outlet1_z5/create_THB ==
  mdot : Inport
  T : Inport  Port=2
  p : Inport  Port=3
  mix : Inport  Port=4
  THB_set_T : carnot/Source/Simple/THB_set_T
  THB_set_mdot : carnot/Source/Simple/THB_set_mdot
  THB_set_mix : Subsystem  InitFcn=load('THB.mat');  mask(set temperature in THB){}
      mask help: Set a variable temperature in the thermo-hydraulic bus.
      mask Help: web(['file:///' fullfile(path_carnot('help'),'THB_set_T.html')],'-helpbrowser')
  THB_set_p : Subsystem  InitFcn=load('THB.mat');  mask(set temperature in THB){}
      mask help: Set a variable temperature in the thermo-hydraulic bus.
      mask Help: web(['file:///' fullfile(path_carnot('help'),'THB_set_T.html')],'-helpbrowser')
  basic_THB : carnot/Basic/Hydraulics/basic_THB  t=20  mdot=0  p=1e5  ID=1  fluid=2  mix=0  dia=0.125  hgt=0
  THB : Outport
  wires:
  T/1 -> THB_set_T/2
  THB_set_mdot/1 -> THB_set_T/1
  mdot/1 -> THB_set_mdot/2
  basic_THB/1 -> THB_set_mdot/1
  THB_set_T/1 -> THB_set_p/1(THB_in)
  THB_set_p/1(THB) -> THB_set_mix/1(THB_in)
  THB_set_mix/1(THB) -> THB/1
  p/1 -> THB_set_p/2(p)
  mix/1 -> THB_set_mix/2(mix)

== system building_EXAMPLE_v1/HVAC pipes/ventilation_outlet1_z6/create_THB ==
  mdot : Inport
  T : Inport  Port=2
  p : Inport  Port=3
  mix : Inport  Port=4
  THB_set_T : carnot/Source/Simple/THB_set_T
  THB_set_mdot : carnot/Source/Simple/THB_set_mdot
  THB_set_mix : Subsystem  InitFcn=load('THB.mat');  mask(set temperature in THB){}
      mask help: Set a variable temperature in the thermo-hydraulic bus.
      mask Help: web(['file:///' fullfile(path_carnot('help'),'THB_set_T.html')],'-helpbrowser')
  THB_set_p : Subsystem  InitFcn=load('THB.mat');  mask(set temperature in THB){}
      mask help: Set a variable temperature in the thermo-hydraulic bus.
      mask Help: web(['file:///' fullfile(path_carnot('help'),'THB_set_T.html')],'-helpbrowser')
  basic_THB : carnot/Basic/Hydraulics/basic_THB  t=20  mdot=0  p=1e5  ID=1  fluid=2  mix=0  dia=0.125  hgt=0
  THB : Outport
  wires:
  T/1 -> THB_set_T/2
  THB_set_mdot/1 -> THB_set_T/1
  mdot/1 -> THB_set_mdot/2
  basic_THB/1 -> THB_set_mdot/1
  THB_set_T/1 -> THB_set_p/1(THB_in)
  THB_set_p/1(THB) -> THB_set_mix/1(THB_in)
  THB_set_mix/1(THB) -> THB/1
  p/1 -> THB_set_p/2(p)
  mix/1 -> THB_set_mix/2(mix)

== system building_EXAMPLE_v1/HVAC pipes/ventilation_outlet1_z7/create_THB ==
  mdot : Inport
  T : Inport  Port=2
  p : Inport  Port=3
  mix : Inport  Port=4
  THB_set_T : carnot/Source/Simple/THB_set_T
  THB_set_mdot : carnot/Source/Simple/THB_set_mdot
  THB_set_mix : Subsystem  InitFcn=load('THB.mat');  mask(set temperature in THB){}
      mask help: Set a variable temperature in the thermo-hydraulic bus.
      mask Help: web(['file:///' fullfile(path_carnot('help'),'THB_set_T.html')],'-helpbrowser')
  THB_set_p : Subsystem  InitFcn=load('THB.mat');  mask(set temperature in THB){}
      mask help: Set a variable temperature in the thermo-hydraulic bus.
      mask Help: web(['file:///' fullfile(path_carnot('help'),'THB_set_T.html')],'-helpbrowser')
  basic_THB : carnot/Basic/Hydraulics/basic_THB  t=20  mdot=0  p=1e5  ID=1  fluid=2  mix=0  dia=0.125  hgt=0
  THB : Outport
  wires:
  T/1 -> THB_set_T/2
  THB_set_mdot/1 -> THB_set_T/1
  mdot/1 -> THB_set_mdot/2
  basic_THB/1 -> THB_set_mdot/1
  THB_set_T/1 -> THB_set_p/1(THB_in)
  THB_set_p/1(THB) -> THB_set_mix/1(THB_in)
  THB_set_mix/1(THB) -> THB/1
  p/1 -> THB_set_p/2(p)
  mix/1 -> THB_set_mix/2(mix)

== system building_EXAMPLE_v1/HVAC pipes/ventilation_outlet1_z8/create_THB ==
  mdot : Inport
  T : Inport  Port=2
  p : Inport  Port=3
  mix : Inport  Port=4
  THB_set_T : carnot/Source/Simple/THB_set_T
  THB_set_mdot : carnot/Source/Simple/THB_set_mdot
  THB_set_mix : Subsystem  InitFcn=load('THB.mat');  mask(set temperature in THB){}
      mask help: Set a variable temperature in the thermo-hydraulic bus.
      mask Help: web(['file:///' fullfile(path_carnot('help'),'THB_set_T.html')],'-helpbrowser')
  THB_set_p : Subsystem  InitFcn=load('THB.mat');  mask(set temperature in THB){}
      mask help: Set a variable temperature in the thermo-hydraulic bus.
      mask Help: web(['file:///' fullfile(path_carnot('help'),'THB_set_T.html')],'-helpbrowser')
  basic_THB : carnot/Basic/Hydraulics/basic_THB  t=20  mdot=0  p=1e5  ID=1  fluid=2  mix=0  dia=0.125  hgt=0
  THB : Outport
  wires:
  T/1 -> THB_set_T/2
  THB_set_mdot/1 -> THB_set_T/1
  mdot/1 -> THB_set_mdot/2
  basic_THB/1 -> THB_set_mdot/1
  THB_set_T/1 -> THB_set_p/1(THB_in)
  THB_set_p/1(THB) -> THB_set_mix/1(THB_in)
  THB_set_mix/1(THB) -> THB/1
  p/1 -> THB_set_p/2(p)
  mix/1 -> THB_set_mix/2(mix)

== system building_EXAMPLE_v1/HVAC pipes/ventilation_outlet1_z9/create_THB ==
  mdot : Inport
  T : Inport  Port=2
  p : Inport  Port=3
  mix : Inport  Port=4
  THB_set_T : carnot/Source/Simple/THB_set_T
  THB_set_mdot : carnot/Source/Simple/THB_set_mdot
  THB_set_mix : Subsystem  InitFcn=load('THB.mat');  mask(set temperature in THB){}
      mask help: Set a variable temperature in the thermo-hydraulic bus.
      mask Help: web(['file:///' fullfile(path_carnot('help'),'THB_set_T.html')],'-helpbrowser')
  THB_set_p : Subsystem  InitFcn=load('THB.mat');  mask(set temperature in THB){}
      mask help: Set a variable temperature in the thermo-hydraulic bus.
      mask Help: web(['file:///' fullfile(path_carnot('help'),'THB_set_T.html')],'-helpbrowser')
  basic_THB : carnot/Basic/Hydraulics/basic_THB  t=20  mdot=0  p=1e5  ID=1  fluid=2  mix=0  dia=0.125  hgt=0
  THB : Outport
  wires:
  T/1 -> THB_set_T/2
  THB_set_mdot/1 -> THB_set_T/1
  mdot/1 -> THB_set_mdot/2
  basic_THB/1 -> THB_set_mdot/1
  THB_set_T/1 -> THB_set_p/1(THB_in)
  THB_set_p/1(THB) -> THB_set_mix/1(THB_in)
  THB_set_mix/1(THB) -> THB/1
  p/1 -> THB_set_p/2(p)
  mix/1 -> THB_set_mix/2(mix)

== system building_EXAMPLE_v1/HVAC pipes/ventilation_pipe_out_1/mix ==
  THB_1 : Inport
  THB_2 : Inport  Port=2
  Add{,1..3} (4 alike) : Sum
  Bus Assignment : BusAssignment  AssignedSignals=Temperature,MassFlow,Pressure,FluidMix
  Bus Selector : BusSelector  OutputSignals=Temperature,MassFlow,Pressure,FluidMix
  Bus Selector2 : BusSelector  OutputSignals=Temperature,MassFlow,Pressure,FluidMix
  Divide : Product  Inputs=*/
  Divide1 : Product  Inputs=*/
  Divide2 : Product  Inputs=*/
  Product{,1..5} (6 alike) : Product
  THB : Outport
  wires:
  Add/1 -> Divide/1  "theta"
  Product1/1 -> Add/2
  Product/1 -> Add/1
  THB_1/1 -> Bus Assignment/1, Bus Selector/1
  Add2/1 -> Divide1/1  "p"
  Product2/1 -> Add2/1
  Product3/1 -> Add2/2
  THB_2/1 -> Bus Selector2/1
  Product4/1 -> Add3/1
  Product5/1 -> Add3/2
  Add3/1 -> Divide2/1  "x"
  Add1/1 -> Divide/2, Divide1/2, Divide2/2, Bus Assignment/3  "massflow"
  Bus Assignment/1 -> THB/1
  Divide2/1 -> Bus Assignment/5
  Divide1/1 -> Bus Assignment/4
  Divide/1 -> Bus Assignment/2
  Bus Selector/1 -> Product/1  "<Temperature>"
  Bus Selector2/1 -> Product1/1  "<Temperature>"
  Bus Selector/3 -> Product2/2  "<Pressure>"
  Bus Selector2/3 -> Product3/2  "<Pressure>"
  Bus Selector/4 -> Product4/2  "<FluidMix>"
  Bus Selector2/4 -> Product5/2  "<FluidMix>"
  Bus Selector/2 -> Product4/1, Product2/1, Add1/1, Product/2  "<MassFlow>"
  Bus Selector2/2 -> Add1/2, Product1/2, Product5/1, Product3/1  "<MassFlow>"

== system building_EXAMPLE_v1/HVAC pipes/ventilation_pipe_out_1/mix1 ==
  THB_1 : Inport
  THB_2 : Inport  Port=2
  Add{,1..3} (4 alike) : Sum
  Bus Assignment : BusAssignment  AssignedSignals=Temperature,MassFlow,Pressure,FluidMix
  Bus Selector : BusSelector  OutputSignals=Temperature,MassFlow,Pressure,FluidMix
  Bus Selector2 : BusSelector  OutputSignals=Temperature,MassFlow,Pressure,FluidMix
  Divide : Product  Inputs=*/
  Divide1 : Product  Inputs=*/
  Divide2 : Product  Inputs=*/
  Product{,1..5} (6 alike) : Product
  THB : Outport
  wires:
  Bus Selector2/2 -> Product3/1, Product5/1, Product1/2, Add1/2  "<MassFlow>"
  Bus Selector/2 -> Product/2, Add1/1, Product2/1, Product4/1  "<MassFlow>"
  Bus Selector2/4 -> Product5/2  "<FluidMix>"
  Bus Selector/4 -> Product4/2  "<FluidMix>"
  Bus Selector2/3 -> Product3/2  "<Pressure>"
  Bus Selector/3 -> Product2/2  "<Pressure>"
  Bus Selector2/1 -> Product1/1  "<Temperature>"
  Bus Selector/1 -> Product/1  "<Temperature>"
  Divide/1 -> Bus Assignment/2
  Divide1/1 -> Bus Assignment/4
  Divide2/1 -> Bus Assignment/5
  Bus Assignment/1 -> THB/1
  Add1/1 -> Bus Assignment/3, Divide2/2, Divide1/2, Divide/2  "massflow"
  Add3/1 -> Divide2/1  "x"
  Product5/1 -> Add3/2
  Product4/1 -> Add3/1
  THB_2/1 -> Bus Selector2/1
  Product3/1 -> Add2/2
  Product2/1 -> Add2/1
  Add2/1 -> Divide1/1  "p"
  THB_1/1 -> Bus Selector/1, Bus Assignment/1
  Product/1 -> Add/1
  Product1/1 -> Add/2
  Add/1 -> Divide/1  "theta"

== system building_EXAMPLE_v1/HVAC pipes/ventilation_pipe_out_1/mix2 ==
  THB_1 : Inport
  THB_2 : Inport  Port=2
  Add{,1..3} (4 alike) : Sum
  Bus Assignment : BusAssignment  AssignedSignals=Temperature,MassFlow,Pressure,FluidMix
  Bus Selector : BusSelector  OutputSignals=Temperature,MassFlow,Pressure,FluidMix
  Bus Selector2 : BusSelector  OutputSignals=Temperature,MassFlow,Pressure,FluidMix
  Divide : Product  Inputs=*/
  Divide1 : Product  Inputs=*/
  Divide2 : Product  Inputs=*/
  Product{,1..5} (6 alike) : Product
  THB : Outport
  wires:
  Add/1 -> Divide/1  "theta"
  Product1/1 -> Add/2
  Product/1 -> Add/1
  THB_1/1 -> Bus Assignment/1, Bus Selector/1
  Add2/1 -> Divide1/1  "p"
  Product2/1 -> Add2/1
  Product3/1 -> Add2/2
  THB_2/1 -> Bus Selector2/1
  Product4/1 -> Add3/1
  Product5/1 -> Add3/2
  Add3/1 -> Divide2/1  "x"
  Add1/1 -> Divide/2, Divide1/2, Divide2/2, Bus Assignment/3  "massflow"
  Bus Assignment/1 -> THB/1
  Divide2/1 -> Bus Assignment/5
  Divide1/1 -> Bus Assignment/4
  Divide/1 -> Bus Assignment/2
  Bus Selector/1 -> Product/1  "<Temperature>"
  Bus Selector2/1 -> Product1/1  "<Temperature>"
  Bus Selector/3 -> Product2/2  "<Pressure>"
  Bus Selector2/3 -> Product3/2  "<Pressure>"
  Bus Selector/4 -> Product4/2  "<FluidMix>"
  Bus Selector2/4 -> Product5/2  "<FluidMix>"
  Bus Selector/2 -> Product4/1, Product2/1, Add1/1, Product/2  "<MassFlow>"
  Bus Selector2/2 -> Add1/2, Product1/2, Product5/1, Product3/1  "<MassFlow>"

== system building_EXAMPLE_v1/HVAC pipes/ventilation_pipe_out_1/mix3 ==
  THB_1 : Inport
  THB_2 : Inport  Port=2
  Add{,1..3} (4 alike) : Sum
  Bus Assignment : BusAssignment  AssignedSignals=Temperature,MassFlow,Pressure,FluidMix
  Bus Selector : BusSelector  OutputSignals=Temperature,MassFlow,Pressure,FluidMix
  Bus Selector2 : BusSelector  OutputSignals=Temperature,MassFlow,Pressure,FluidMix
  Divide : Product  Inputs=*/
  Divide1 : Product  Inputs=*/
  Divide2 : Product  Inputs=*/
  Product{,1..5} (6 alike) : Product
  THB : Outport
  wires:
  Bus Selector2/2 -> Product3/1, Product5/1, Product1/2, Add1/2  "<MassFlow>"
  Bus Selector/2 -> Product/2, Add1/1, Product2/1, Product4/1  "<MassFlow>"
  Bus Selector2/4 -> Product5/2  "<FluidMix>"
  Bus Selector/4 -> Product4/2  "<FluidMix>"
  Bus Selector2/3 -> Product3/2  "<Pressure>"
  Bus Selector/3 -> Product2/2  "<Pressure>"
  Bus Selector2/1 -> Product1/1  "<Temperature>"
  Bus Selector/1 -> Product/1  "<Temperature>"
  Divide/1 -> Bus Assignment/2
  Divide1/1 -> Bus Assignment/4
  Divide2/1 -> Bus Assignment/5
  Bus Assignment/1 -> THB/1
  Add1/1 -> Bus Assignment/3, Divide2/2, Divide1/2, Divide/2  "massflow"
  Add3/1 -> Divide2/1  "x"
  Product5/1 -> Add3/2
  Product4/1 -> Add3/1
  THB_2/1 -> Bus Selector2/1
  Product3/1 -> Add2/2
  Product2/1 -> Add2/1
  Add2/1 -> Divide1/1  "p"
  THB_1/1 -> Bus Selector/1, Bus Assignment/1
  Product/1 -> Add/1
  Product1/1 -> Add/2
  Add/1 -> Divide/1  "theta"
